simulink model "pfb4t11_bb"  (Simulink 8.0)
settings: Solver=VariableStepDiscrete  SolverMode=SingleTasking  StartTime=0.0  StopTime=10.0  RelTol=1e-3
undefined symbols (not defined in the file or in its folder): pfb_coeff_gen_calc
libraries: xbsIndex_r4 x700, casper_library_delays x96, casper_library_pfbs x2
(part 1 of 9)
settings Model: Creator=ptcs  LastModifiedBy=ptcs
settings DataIOCC: SignalLoggingSaveFormat=ModelDataLogs
settings OptimizationCC: InlineParams=on
settings DebuggingCC: FcnCallInpInsideContextMsg=EnableAllAsWarning

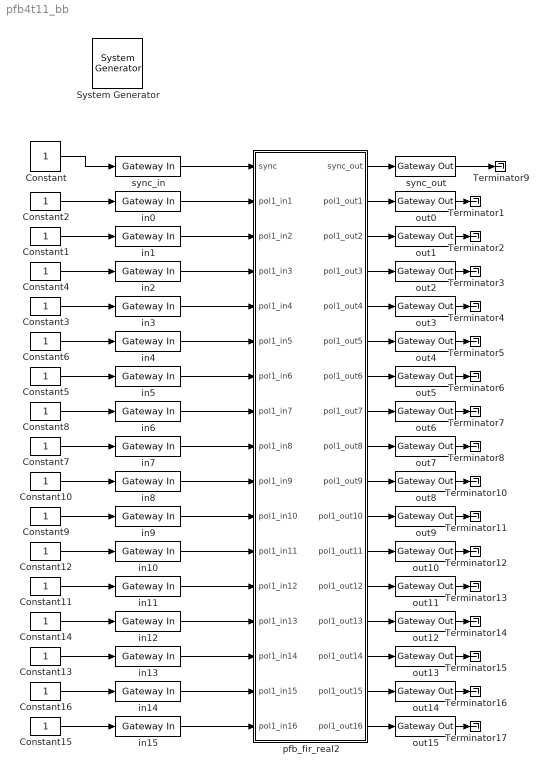
== system pfb4t11_bb ==
  " System Generator" : xbsIndex_r4/ System Generator  Tag=genX  xilinxfamily=virtex6  part=xc6vsx475t  speed=-1  package=ff1759  synthesis_tool=XST  clock_wrapper=Clock Enables  directory=./pfb4t11_bb  proj_type=Project Navigator  Synth_file=XST Defaults  Impl_file=ISE Defaults  testbench=off  simulink_period=1  sysclk_period=10  dcm_input_clock_period=10  incr_netlist=off  trim_vbits=Everywhere in SubSystem  dbl_ovrd=According to Block Masks  core_generation=According to Block Masks  run_coregen=off  deprecated_control=off  eval_field=0  block_type=sysgen
  Constant{,1..16} (17 alike) : Constant  SampleTime=1
  Terminator{1..17} (17 alike) : Terminator
  in{0..15} (16 alike) : xbsIndex_r4/Gateway In  gui_display_data_type=Fixed-point  arith_type="Signed  (2's comp)"  n_bits=8  bin_pt=7  preci_type=Single  exp_width=8  frac_width=24  quantization=Truncate  overflow=Wrap  period=1  dbl_ovrd=off  timing_constraint=None  locs_specified=off  LOCs={}  UseAsADC=off  ADCChannel='1'  inherit_from_input=off  hdl_port=on  block_type=gatewayin
  out{0..15} (16 alike) : xbsIndex_r4/Gateway Out  inherit_from_input=off  hdl_port=on  timing_constraint=None  locs_specified=off  LOCs={}  UseAsDAC=off  DACChannel='1'  block_type=gatewayout
  pfb_fir_real2 : Subsystem  Tag=casper:pfb_fir_real  AncestorBlock=casper_library_pfbs/pfb_fir_real  mask(pfb_fir_real){PFBSize=11, TotalTaps=4, WindowType=hamming, n_inputs=4, MakeBiplex=off, BitWidthIn=8, BitWidthOut=18, CoeffBitWidth=18, CoeffDistMem=off, add_latency=1, mult_latency=2, bram_latency=2, fan_latency=1, conv_latency=1, quantization=Round  (unbiased: Even Values), fwidth=1, mult_spec=2, adder_folding=on, adder_imp=Fabric, coeffs_share=off}
      mask prompts: PFBSize "Size of PFB: (2^? pnts)"; TotalTaps "Total Number of Taps:"; WindowType "Windowing Function:"; n_inputs "Number of Simultaneous Inputs: (2^?)"; MakeBiplex "Make Biplex?"; BitWidthIn "Input Bitwidth:"; BitWidthOut "Output Bitwidth:"; CoeffBitWidth "Coefficient Bitwidth:"; CoeffDistMem "Use Distributed Memory for Coeffs"; add_latency "Add Latency"; mult_latency "Mult Latency"; bram_latency "BRAM Latency"; fan_latency "Fanout latency"; conv_latency "Convert latency"; quantization "Quantization Behavior"; fwidth "Bin Width Scaling (normal=1)"; mult_spec "Multiplier specification (0=core, 1=embedded, 2=behavioural) (left=1st tap, or just one value)"; adder_folding "Fold adders into DSPs"; adder_imp "Adder implementation"; coeffs_share "Share coefficients between polarisations (use less BRAM)?"
      mask help:
      | Fold adders into DSPs: Causes adders to be absorbed into DSP blocks (supported in Virtex5)
      | Adder implementation: Cores using Fabric or DSP48 or behavioral HDL
      mask init:
      | pfb_fir_real_init(gcb, ...
      |     'PFBSize', PFBSize, ...
      |     'TotalTaps', TotalTaps, ...
      |     'WindowType', WindowType, ...
      |     'n_inputs', n_inputs, ...
      |     'MakeBiplex', MakeBiplex, ...
      |     'BitWidthIn', BitWidthIn, ...
      |     'BitWidthOut', BitWidthOut, ...
      |     'CoeffBitWidth', CoeffBitWidth, ...
      |     'CoeffDistMem', CoeffDistMem, ...
      |     'add_latency', add_latency, ...
      |     'mult_latency', mult_latency, ...
      |     'bram_latency', bram_latency, ...
      |     'fan_latency', fan_latency, ...
      |     'conv_latency', conv_latency, ...
      |     'quantization', quantization, ...
      |     'fwidth', fwidth, ...
      |     'mult_spec', mult_spec, ...
      |     'adder_folding', adder_folding, ...
      |     'adder_imp', adder_imp, ...
      |     'coeffs_share', coeffs_share);
      settings: AttributesFormatString=taps=4, add_latency=1
      mask Help: eval('xlWeb(''http://casper.berkeley.edu/wiki/Pfb_fir_real'')')
      mask Callback TotalTaps:
      | %num_taps = eval(get_param(gcb, 'TotalTaps'));
      | %old_vec = eval(get_param(gcb, 'mult_spec'));=-0l
      | 
      | %vec = 2.*ones(1,num_taps);
      | %old_size = length(old_vec);
      | 
      | %if(old_size <= num_taps),
      | %    new_size = old_size;
      | %else,
      | %    new_size = num_taps;
      | %end
      | 
      | %for n = 1:new_size, vec(n) = old_vec(n); end
      | %set_param(gcb, 'mult_spec', mat2str(vec));
      mask TypeOptions WindowType: bartlett | barthannwin | blackman | blackmanharris | bohamwin | chebwin | flattopwin | gausswin | hamming | hann | kaiser | nuttallwin | parzenwin | rectwin | tukeywin | triang | userwindow
      mask TypeOptions quantization: Truncate | Round  (unbiased: +/- Inf) | Round  (unbiased: Even Values)
      mask TypeOptions adder_imp: Behavioral | Fabric | DSP48
  sync_in : xbsIndex_r4/Gateway In  gui_display_data_type=Boolean  arith_type=Boolean  n_bits=16  bin_pt=14  preci_type=Single  exp_width=8  frac_width=24  quantization="Round  (unbiased: +/- Inf)"  overflow=Saturate  period=1  dbl_ovrd=off  timing_constraint=None  locs_specified=off  LOCs={}  UseAsADC=off  ADCChannel='1'  inherit_from_input=off  hdl_port=on  block_type=gatewayin
  sync_out : xbsIndex_r4/Gateway Out  inherit_from_input=off  hdl_port=on  timing_constraint=None  locs_specified=off  LOCs={}  UseAsDAC=off  DACChannel='1'  block_type=gatewayout
  wires:
  Constant/1 -> sync_in/1
  Constant2/1 -> in0/1
  out0/1 -> Terminator1/1
  sync_out/1 -> Terminator9/1
  Constant1/1 -> in1/1
  Constant4/1 -> in2/1
  Constant3/1 -> in3/1
  Constant6/1 -> in4/1
  Constant5/1 -> in5/1
  Constant8/1 -> in6/1
  Constant7/1 -> in7/1
  Constant10/1 -> in8/1
  Constant9/1 -> in9/1
  Constant12/1 -> in10/1
  Constant11/1 -> in11/1
  Constant14/1 -> in12/1
  Constant13/1 -> in13/1
  Constant16/1 -> in14/1
  Constant15/1 -> in15/1
  sync_in/1 -> pfb_fir_real2/1(sync)
  in0/1 -> pfb_fir_real2/2(pol1_in1)
  in1/1 -> pfb_fir_real2/3(pol1_in2)
  in2/1 -> pfb_fir_real2/4(pol1_in3)
  in3/1 -> pfb_fir_real2/5(pol1_in4)
  in4/1 -> pfb_fir_real2/6(pol1_in5)
  in5/1 -> pfb_fir_real2/7(pol1_in6)
  in6/1 -> pfb_fir_real2/8(pol1_in7)
  in7/1 -> pfb_fir_real2/9(pol1_in8)
  in8/1 -> pfb_fir_real2/10(pol1_in9)
  in9/1 -> pfb_fir_real2/11(pol1_in10)
  in10/1 -> pfb_fir_real2/12(pol1_in11)
  in11/1 -> pfb_fir_real2/13(pol1_in12)
  in12/1 -> pfb_fir_real2/14(pol1_in13)
  in13/1 -> pfb_fir_real2/15(pol1_in14)
  in14/1 -> pfb_fir_real2/16(pol1_in15)
  in15/1 -> pfb_fir_real2/17(pol1_in16)
  pfb_fir_real2/1(sync_out) -> sync_out/1
  out1/1 -> Terminator2/1
  out2/1 -> Terminator3/1
  out3/1 -> Terminator4/1
  out4/1 -> Terminator5/1
  out5/1 -> Terminator6/1
  out6/1 -> Terminator7/1
  out7/1 -> Terminator8/1
  out8/1 -> Terminator10/1
  out9/1 -> Terminator11/1
  out10/1 -> Terminator12/1
  out11/1 -> Terminator13/1
  out12/1 -> Terminator14/1
  out13/1 -> Terminator15/1
  out14/1 -> Terminator16/1
  out15/1 -> Terminator17/1
  pfb_fir_real2/2(pol1_out1) -> out0/1
  pfb_fir_real2/3(pol1_out2) -> out1/1
  pfb_fir_real2/4(pol1_out3) -> out2/1
  pfb_fir_real2/5(pol1_out4) -> out3/1
  pfb_fir_real2/6(pol1_out5) -> out4/1
  pfb_fir_real2/7(pol1_out6) -> out5/1
  pfb_fir_real2/8(pol1_out7) -> out6/1
  pfb_fir_real2/9(pol1_out8) -> out7/1
  pfb_fir_real2/10(pol1_out9) -> out8/1
  pfb_fir_real2/11(pol1_out10) -> out9/1
  pfb_fir_real2/12(pol1_out11) -> out10/1
  pfb_fir_real2/13(pol1_out12) -> out11/1
  pfb_fir_real2/14(pol1_out13) -> out12/1
  pfb_fir_real2/15(pol1_out14) -> out13/1
  pfb_fir_real2/16(pol1_out15) -> out14/1
  pfb_fir_real2/17(pol1_out16) -> out15/1
